simulink library "Teleop_lib"  (R2023b)
settings: Solver=VariableStepAuto  StartTime=0.0  StopTime=10.0  RelTol=1e-3
settings Model: Creator=FIRSTMentor  LastModifiedBy=ander

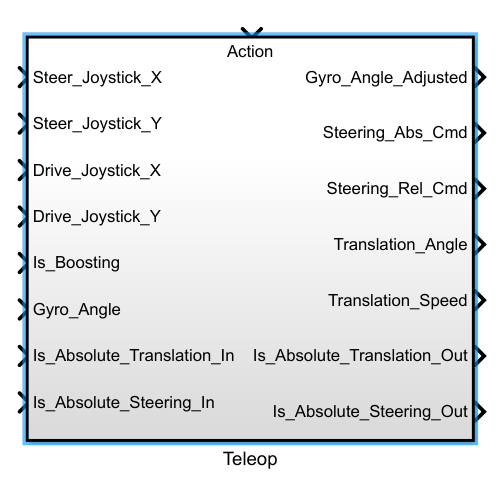
[thumbnail: Simulink's stored preview of the top-level diagram]
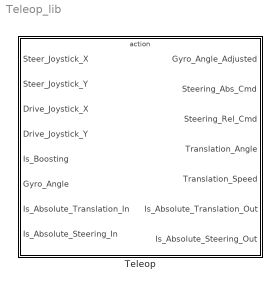
== system Teleop_lib ==
  Teleop : Subsystem  TreatAsAtomicUnit=on

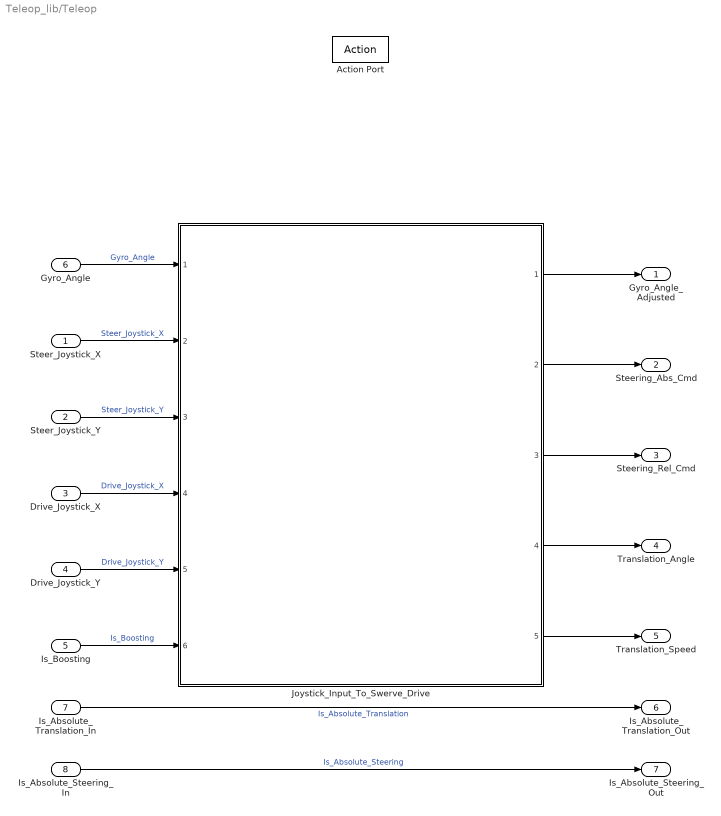
== system Teleop_lib/Teleop ==
  Steer_Joystick_X : Inport
  Steer_Joystick_Y : Inport  Port=2
  Drive_Joystick_X : Inport  Port=3
  Drive_Joystick_Y : Inport  Port=4
  Is_Boosting : Inport  Port=5
  Gyro_Angle : Inport  Port=6
  Is_Absolute_Translation_In : Inport  Port=7
  Is_Absolute_Steering_In : Inport  Port=8
  Action Port : ActionPort
  Joystick_Input_To_Swerve_Drive : Subsystem  ReferencedSubsystem=Joystick_Input_To_Swerve_Drive_sub
  Gyro_Angle_Adjusted : Outport
  Steering_Abs_Cmd : Outport  Port=2
  Steering_Rel_Cmd : Outport  Port=3
  Translation_Angle : Outport  Port=4
  Translation_Speed : Outport  Port=5
  Is_Absolute_Translation_Out : Outport  Port=6
  Is_Absolute_Steering_Out : Outport  Port=7
  wires:
  Steer_Joystick_X/1 -> Joystick_Input_To_Swerve_Drive/2  "Steer_Joystick_X"
  Steer_Joystick_Y/1 -> Joystick_Input_To_Swerve_Drive/3  "Steer_Joystick_Y"
  Drive_Joystick_X/1 -> Joystick_Input_To_Swerve_Drive/4  "Drive_Joystick_X"
  Drive_Joystick_Y/1 -> Joystick_Input_To_Swerve_Drive/5  "Drive_Joystick_Y"
  Joystick_Input_To_Swerve_Drive/1 -> Gyro_Angle_Adjusted/1
  Joystick_Input_To_Swerve_Drive/2 -> Steering_Abs_Cmd/1
  Joystick_Input_To_Swerve_Drive/3 -> Steering_Rel_Cmd/1
  Joystick_Input_To_Swerve_Drive/4 -> Translation_Angle/1
  Joystick_Input_To_Swerve_Drive/5 -> Translation_Speed/1
  Is_Absolute_Translation_In/1 -> Is_Absolute_Translation_Out/1  "Is_Absolute_Translation"
  Is_Absolute_Steering_In/1 -> Is_Absolute_Steering_Out/1  "Is_Absolute_Steering"
  Gyro_Angle/1 -> Joystick_Input_To_Swerve_Drive/1  "Gyro_Angle"
  Is_Boosting/1 -> Joystick_Input_To_Swerve_Drive/6  "Is_Boosting"
